simulink model "PID_Controllers"  (R2021a)
settings: Solver=VariableStepAuto  StartTime=0.0  StopTime=10.0  RelTol=1e-3
values from neighbouring files (symbols this model uses):
  A = 0.0085    [distiller_controller_state_space_model.m]
  A_rad = 1.01    [distiller_controller_state_space_model.m]
  c = 4200    [distiller_controller_state_space_model.m]
  h_conv = 50    [distiller_controller_state_space_model.m]
  m_coolant = 25    [distiller_controller_state_space_model.m]
  m_still = 10    [distiller_controller_state_space_model.m]
libraries: pid_lib x4
settings Model: Creator=Intuito_PC  LastModifiedBy=Intuito_PC

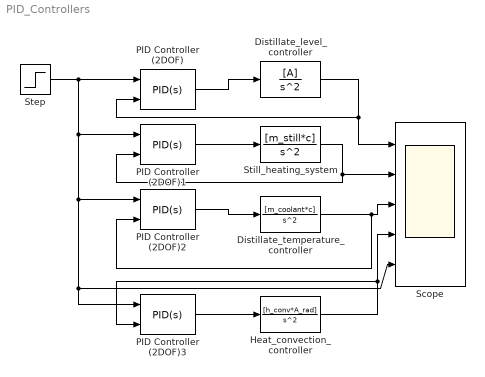
== system PID_Controllers ==
  Distillate_level_controller : TransferFcn  Numerator=[A]  Denominator=[1, 0, 0]
  Distillate_temperature_controller : TransferFcn  Numerator=[m_coolant*c]  Denominator=[1, 0, 0]
  Heat_convection_controller : TransferFcn  Numerator=[h_conv*A_rad]  Denominator=[1, 0, 0]
  PID Controller (2DOF){,1..3} (4 alike) : pid_lib/PID Controller (2DOF)  Controller=PID  Form=Parallel  TimeDomain=Continuous-time  UseExternalTs=off  SampleTime=-1  IntegratorMethod=Forward Euler  FilterMethod=Forward Euler  ControllerParametersSource=internal  P=1  I=1  D=0  UseFilter=on  N=100  b=1  c=1  TunerSelectOption=Transfer Function Based (PID Tuner App)  InitialConditionSource=internal  InitialConditionForIntegrator=0  InitialConditionForFilter=0  DifferentiatorICPrevScaledInput=0  ExternalReset=none  TrackingMode=off  Kt=1  LimitOutput=off  SatLimitsSource=internal  UpperSaturationLimit=inf  LowerSaturationLimit=-inf  LinearizeAsGain=on  AntiWindupMode=none  Kb=1  POutMin=[]  POutMax=[]  IOutMin=[]  IOutMax=[]  DOutMin=[]  DOutMax=[]  NOutMin=[]  NOutMax=[]  bOutMin=[]  bOutMax=[]  cOutMin=[]  cOutMax=[]  SumOutMin=[]  SumOutMax=[]  SaturationOutMin=[]  SaturationOutMax=[]  PParamMin=[]  PParamMax=[]  IParamMin=[]  IParamMax=[]  DParamMin=[]  DParamMax=[]  NParamMin=[]  NParamMax=[]  bParamMin=[]  bParamMax=[]  cParamMin=[]  cParamMax=[]  KbParamMin=[]  KbParamMax=[]  KtParamMin=[]  KtParamMax=[]  KbOutMin=[]  KbOutMax=[]  KtOutMin=[]  KtOutMax=[]  IntegratorOutMin=[]  IntegratorOutMax=[]  FilterOutMin=[]  FilterOutMax=[]  SumI1OutMin=[]  SumI1OutMax=[]  SumI2OutMin=[]  SumI2OutMax=[]  SumI3OutMin=[]  SumI3OutMax=[]  SumI4OutMin=[]  SumI4OutMax=[]  SumDOutMin=[]  SumDOutMax=[]  Sum1OutMin=[]  Sum1OutMax=[]  Sum2OutMin=[]  Sum2OutMax=[]  Sum3OutMin=[]  Sum3OutMax=[]  DifferentiatorOutMin=[]  DifferentiatorOutMax=[]  FilterDiffOutCoefMin=[]  FilterDiffOutCoefMax=[]  ReciprocalOutMin=[]  ReciprocalOutMax=[]  SumDenOutMin=[]  SumDenOutMax=[]  SumNumOutMin=[]  SumNumOutMax=[]  DivideOutMin=[]  DivideOutMax=[]  UdiffTsProdOutMin=[]  UdiffTsProdOutMax=[]  NTsProdOutMin=[]  NTsProdOutMax=[]  UintegralTsProdOutMin=[]  UintegralTsProdOutMax=[]  UngainTsProdOutMin=[]  UngainTsProdOutMax=[]  IntegratorContinuousStateAttributes=''  IntegratorStateMustResolveToSignalObject=off  IntegratorRTWStateStorageClass=Auto  FilterContinuousStateAttributes=''  FilterStateMustResolveToSignalObject=off  FilterRTWStateStorageClass=Auto  ParallelPVariant=InternalParameters  IdealPVariant=Disabled  IVariant=InternalParameters  DVariant=InternalParameters  bVariant=InternalParameters  cVariant=InternalParameters  IntegratorVariant=Continuous  SatVariant=Disabled  AWVariant=Passthrough  PCopyVariant=Disabled  TRVariant=Disabled  FdbkBlocksVariant=Forward  IdealPFdbkVariant=Disabled  SatFdbkVariant=Disabled  DerivativeFilterVariant=ContFilter  NVariant=InternalParameters  NCopyVariant=Disabled  FilterICVariant=InternalICsFilter  IntegratorICVariant=InternalICs  ExternalResetVariant=Disabled  TRSumVariant=Passthrough  SumFdbkVariant=Disabled  SumVariant=Sum_PID  TsampFilterVariant=InternalTs  TsampNgainVariant=Passthrough  TsampIntegralVariant=Passthrough  ExternalSaturationOutDataTypeStr=Inherit: Same as second input
      settings: SourceProductBaseCode=SL
  Scope : Scope  NumInputPorts=5
  Step : Step  SampleTime=0
  Still_heating_system : TransferFcn  Numerator=[m_still*c]  Denominator=[1, 0, 0]
  wires:
  Distillate_level_controller/1 -> Scope/1, PID Controller (2DOF)/2
  Still_heating_system/1 -> PID Controller (2DOF)1/2, Scope/2
  Distillate_temperature_controller/1 -> PID Controller (2DOF)2/2, Scope/3
  Heat_convection_controller/1 -> PID Controller (2DOF)3/2, Scope/4
  PID Controller (2DOF)/1 -> Distillate_level_controller/1
  PID Controller (2DOF)1/1 -> Still_heating_system/1
  PID Controller (2DOF)2/1 -> Distillate_temperature_controller/1
  PID Controller (2DOF)3/1 -> Heat_convection_controller/1
  Step/1 -> PID Controller (2DOF)3/1, Scope/5, PID Controller (2DOF)2/1, PID Controller (2DOF)1/1, PID Controller (2DOF)/1
